simulink model "system model"  (R2015b)
settings: Solver=VariableStepAuto  StartTime=0.0  StopTime=1.5  RelTol=1e-3
values from neighbouring files (symbols this model uses):
  a = [20000000 44020000 28944000 3748900 1672280 352676 189124 37657 30]    [system specifications.m]
  b = [100000 130100 30130 30 0 0]    [system specifications.m]
  K = acker (A,B,Pc)    [system specifications.m]
  L = acker (A',C',Po)'    [system specifications.m]
undefined symbols (not defined in the file or in its folder): A, B, C, D
settings Model: Creator=Олег  LastModifiedBy=Олег

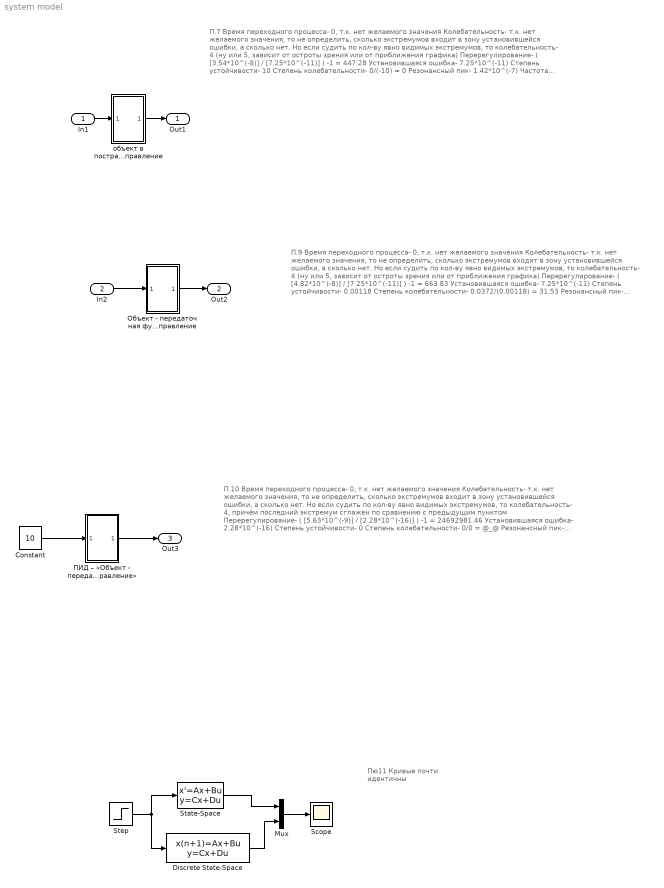
== system system model ==
  note: Пю11
      | Кривые почти идентичны
  note: П.10
      | Время переходного процесса- 0, т.к. нет желаемого значения
      |
      | Колебательность- т.к. нет желаемого значения, то не определить, сколько экстремумов
      | входит в зону установившейся ошибки, а сколько нет. Но если судить по кол-ву явно видимых
      | экстремумов, то колебательность- 4, причём последний экстремум сглажен по сравнению с предыдущим пунктом
      |
      | Перерегулирование- ( [5.63*10^(-9)] / [2.28*10^(-16)] ) -1 = 24692981.46
      |
      | Установившаяся ошибка- 2.28*10^(-16)
      |
      | Степень устойчивости-  0
      |
      | Степень колебательности- 0/0 = @_@
      |
      | Резонансный пик- 1.66*10^(-8)
      |
      | Частота пропускания- 25.8 рад/с
      |
      | Частота среза- отсутствует, т.к. ЛАЧХ не пересекает отметку 0
  note: П.9
      | Время переходного процесса- 0, т.к. нет желаемого значения
      |
      | Колебательность- т.к. нет желаемого значения, то не определить, сколько экстремумов
      | входит в зону установившейся ошибки, а сколько нет. Но если судить по кол-ву явно видимых
      | экстремумов, то колебательность- 4 (ну или 5, зависит от остроты зрения или от приближения графика)
      |
      | Перерегулирование- ( [4.82*10^(-8)] / [7.25*10^(-11)] ) -1 = 663.83
      |
      | Установившаяся ошибка- 7.25*10^(-11)
      |
      | Степень устойчивости-  0.00118
      |
      | Степень колебательности- 0.0372/(0.00118) = 31.53
      |
      | Резонансный пик- 1.42*10^(-7)
      |
      | Частота пропускания- 27.4 рад/с
      |
      | Частота среза- отсутствует, т.к. ЛАЧХ не пересекает отметку 0
  note: П.7
      | Время переходного процесса- 0, т.к. нет желаемого значения
      |
      | Колебательность- т.к. нет желаемого значения, то не определить, сколько экстремумов
      | входит в зону установившейся ошибки, а сколько нет. Но если судить по кол-ву явно видимых
      | экстремумов, то колебательность- 4 (ну или 5, зависит от остроты зрения или от приближения графика)
      |
      | Перерегулирование- ( [3.54*10^(-8)] / [7.25*10^(-11)] ) -1 = 447.28
      |
      | Установившаяся ошибка- 7.25*10^(-11)
      |
      | Степень устойчивости-  10
      |
      | Степень колебательности- 0/(-10) = 0
      |
      | Резонансный пик- 1.42*10^(-7)
      |
      | Частота пропускания- 27.4 рад/с
      |
      | Частота среза- отсутствует, т.к. ЛАЧХ не пересекает отметку 0
  In1 : Inport
  In2 : Inport  Port=2
  Constant : Constant  Value=10
  Discrete State-Space : DiscreteStateSpace  A=(A*0.001+eye(8))  B=B*0.001  C=C  D=D  SampleTime=0.001
  Mux : Mux  Inputs=2
  Scope : Scope
  State-Space : StateSpace  A=A  B=B  C=C  D=D  X0=0
  Step : Step  Time=0.5  SampleTime=0
  "Объект - передаточная функция, наблюдатель полного порядка-модальное управление" : Subsystem
  "ПИД – «Объект - передаточную функцию, наблюдатель полного порядка-модальное управление»" : Subsystem
  объект в постранстве состояний - модальное управление : Subsystem
  Out1 : Outport
  Out2 : Outport  Port=2
  Out3 : Outport  Port=3
  wires:
  In1/1 -> объект в постранстве состояний - модальное управление/1(In1)
  объект в постранстве состояний - модальное управление/1(Out1) -> Out1/1
  In2/1 -> "Объект - передаточная функция, наблюдатель полного порядка-модальное управление"/1(In1)
  "Объект - передаточная функция, наблюдатель полного порядка-модальное управление"/1(Out1) -> Out2/1
  Step/1 -> State-Space/1, Discrete State-Space/1
  Mux/1 -> Scope/1
  Discrete State-Space/1 -> Mux/2
  State-Space/1 -> Mux/1
  Constant/1 -> "ПИД – «Объект - передаточную функцию, наблюдатель полного порядка-модальное управление»"/1(In1)
  "ПИД – «Объект - передаточную функцию, наблюдатель полного порядка-модальное управление»"/1(Out1) -> Out3/1

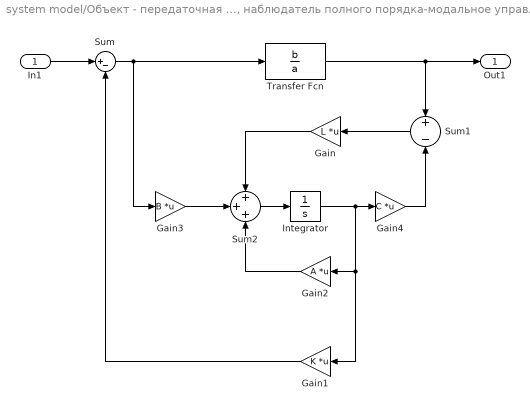
== system system model/Объект - передаточная функция, наблюдатель полного порядка-модальное управление ==
  In1 : Inport
  Gain : Gain  Gain=L  Multiplication=Matrix(K*u)
  Gain1 : Gain  Gain=K  Multiplication=Matrix(K*u)
  Gain2 : Gain  Gain=A  Multiplication=Matrix(K*u)
  Gain3 : Gain  Gain=B  Multiplication=Matrix(K*u)
  Gain4 : Gain  Gain=C  Multiplication=Matrix(K*u)
  Integrator : Integrator
  Sum : Sum  Inputs=|+-
  Sum1 : Sum  Inputs=+|-
  Sum2 : Sum  Inputs=+++
  Transfer Fcn : TransferFcn  Numerator=b  Denominator=a
  Out1 : Outport
  wires:
  In1/1 -> Sum/1
  Gain/1 -> Sum2/1
  Gain1/1 -> Sum/2
  Gain3/1 -> Sum2/2
  Gain2/1 -> Sum2/3
  Sum/1 -> Gain3/1, Transfer Fcn/1
  Sum2/1 -> Integrator/1
  Sum1/1 -> Gain/1
  Integrator/1 -> Gain2/1, Gain1/1, Gain4/1
  Gain4/1 -> Sum1/2
  Transfer Fcn/1 -> Out1/1, Sum1/1

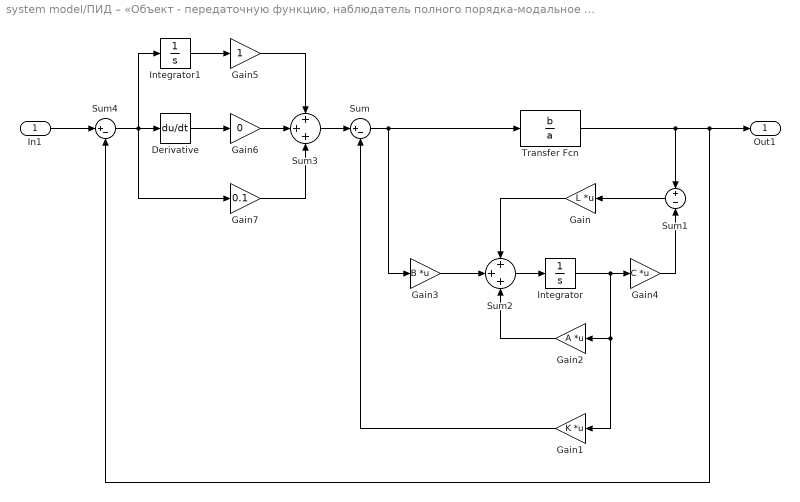
== system system model/ПИД – «Объект - передаточную функцию, наблюдатель полного порядка-модальное управление» ==
  In1 : Inport
  Derivative : Derivative
  Gain : Gain  Gain=L  Multiplication=Matrix(K*u)
  Gain1 : Gain  Gain=K  Multiplication=Matrix(K*u)
  Gain2 : Gain  Gain=A  Multiplication=Matrix(K*u)
  Gain3 : Gain  Gain=B  Multiplication=Matrix(K*u)
  Gain4 : Gain  Gain=C  Multiplication=Matrix(K*u)
  Gain5 : Gain
  Gain6 : Gain  Gain=0
  Gain7 : Gain  Gain=0.1
  Integrator : Integrator
  Integrator1 : Integrator
  Sum : Sum  Inputs=|+-
  Sum1 : Sum  Inputs=+|-
  Sum2 : Sum  Inputs=+++
  Sum3 : Sum  Inputs=+++
  Sum4 : Sum  Inputs=|+-
  Transfer Fcn : TransferFcn  Numerator=b  Denominator=a
  Out1 : Outport
  wires:
  Gain3/1 -> Sum2/2
  Gain1/1 -> Sum/2
  Gain/1 -> Sum2/1
  Gain7/1 -> Sum3/3
  Derivative/1 -> Gain6/1
  Sum4/1 -> Gain7/1, Integrator1/1, Derivative/1
  In1/1 -> Sum4/1
  Transfer Fcn/1 -> Out1/1, Sum4/2, Sum1/1
  Sum3/1 -> Sum/1
  Gain6/1 -> Sum3/2
  Sum/1 -> Gain3/1, Transfer Fcn/1
  Integrator1/1 -> Gain5/1
  Integrator/1 -> Gain2/1, Gain1/1, Gain4/1
  Gain4/1 -> Sum1/2
  Sum1/1 -> Gain/1
  Gain5/1 -> Sum3/1
  Gain2/1 -> Sum2/3
  Sum2/1 -> Integrator/1

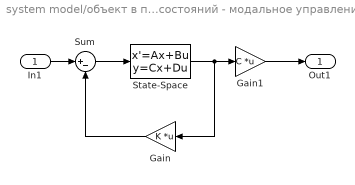
== system system model/объект в постранстве состояний - модальное управление ==
  In1 : Inport
  Gain : Gain  Gain=K  Multiplication=Matrix(K*u)
  Gain1 : Gain  Gain=C  Multiplication=Matrix(K*u)
  State-Space : StateSpace  A=A  B=B  C=eye(8)  D=zeros(8,1)  X0=0
  Sum : Sum  Inputs=|+-
  Out1 : Outport
  wires:
  State-Space/1 -> Gain/1, Gain1/1
  Sum/1 -> State-Space/1
  In1/1 -> Sum/1
  Gain1/1 -> Out1/1
  Gain/1 -> Sum/2
